simulink model "model2"  (R2018b)
settings: Solver=VariableStepAuto  StartTime=0.0  StopTime=8  RelTol=1e-3
settings Model: Creator=HYJ  LastModifiedBy=HYJ
settings CodeAppCC: StateflowObjectComments=on

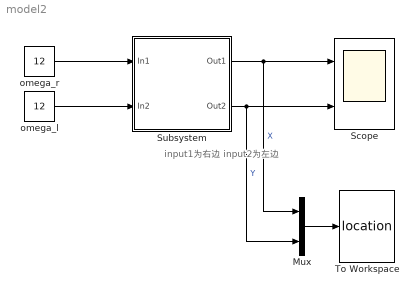
== system model2 ==
  note: input1为右边
      | input2为左边
  Mux : Mux  Inputs=2
  Scope : Scope  NumInputPorts=2
  Subsystem : Subsystem  mask{rear_wheel_radius=0.3, wheelchair_width=0.8}
  To Workspace : ToWorkspace  VariableName=location  SampleTime=-1
      settings: Save2DSignal=2-D array (concatenate along first dimension)
  omega_l : Constant  Value=12
  omega_r : Constant  Value=12
  wires:
  Subsystem/1(Out1) -> Mux/1, Scope/1  "X"
  Subsystem/2(Out2) -> Mux/2, Scope/2  "Y"
  omega_r/1 -> Subsystem/1(In1)
  omega_l/1 -> Subsystem/2(In2)
  Mux/1 -> To Workspace/1

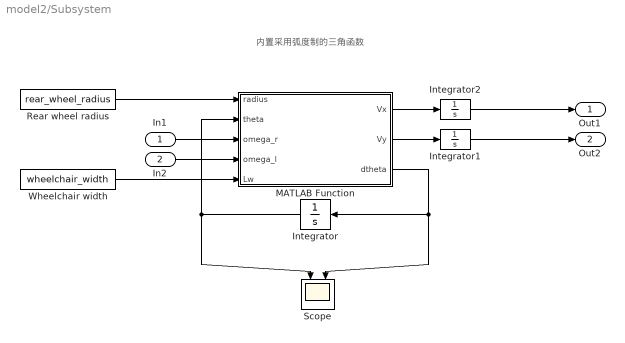
== system model2/Subsystem ==
  note: 内置采用弧度制的三角函数
  In1 : Inport
  In2 : Inport  Port=2
  Integrator : Integrator
  Integrator1 : Integrator
  Integrator2 : Integrator
  MATLAB Function : MATLAB Function  TreatAsAtomicUnit=on
  Rear wheel radius : Constant  Value=rear_wheel_radius
  Scope : Scope  NumInputPorts=2
  Wheelchair width : Constant  Value=wheelchair_width
  Out1 : Outport
  Out2 : Outport  Port=2
  wires:
  MATLAB Function/2(Vy) -> Integrator1/1
  MATLAB Function/1(Vx) -> Integrator2/1
  Rear wheel radius/1 -> MATLAB Function/1(radius)
  MATLAB Function/3(dtheta) -> Scope/2, Integrator/1
  In1/1 -> MATLAB Function/3(omega_r)
  In2/1 -> MATLAB Function/4(omega_l)
  Wheelchair width/1 -> MATLAB Function/5(Lw)
  Integrator/1 -> MATLAB Function/2(theta), Scope/1
  Integrator2/1 -> Out1/1
  Integrator1/1 -> Out2/1

== matlab function model2/Subsystem/MATLAB Function ==
  data: Vx output; radius input; Vy output; theta input; omega_r input; omega_l input; Lw input; dtheta output
function [Vx, Vy, dtheta] = MPW_main(radius, theta, omega_r, omega_l, Lw)

Vx = 0.5 * radius * cos(theta) * (omega_r + omega_l);
Vy = 0.5 * radius * sin(theta) * (omega_r + omega_l);
dtheta = 2 * radius * ((omega_r/Lw) - (omega_l/Lw));

end
